simulink model "LQR-1"  (R2018a)
settings: Solver=VariableStepAuto  StartTime=0.0  StopTime=10.0  RelTol=1e-3
settings Model: Creator=86153  LastModifiedBy=86153

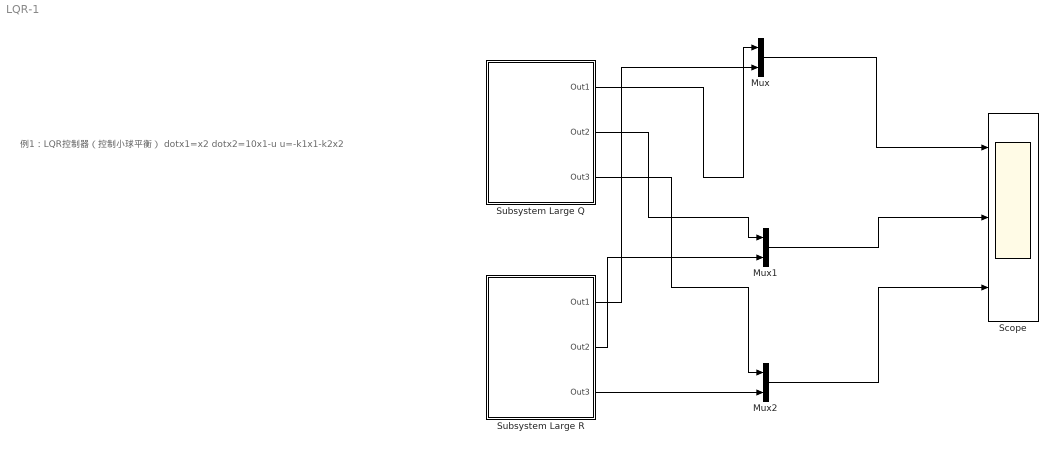
== system LQR-1 ==
  note: 例1：LQR控制器（控制小球平衡）
      | dotx1=x2
      | dotx2=10x1-u
      | u=-k1x1-k2x2
  Mux : Mux  Inputs=2
  Mux1 : Mux  Inputs=2
  Mux2 : Mux  Inputs=2
  Scope : Scope  NumInputPorts=3
  Subsystem Large Q : Subsystem
  Subsystem Large R : Subsystem
  wires:
  Subsystem Large Q/1(Out1) -> Mux/1
  Subsystem Large Q/2(Out2) -> Mux1/1
  Subsystem Large Q/3(Out3) -> Mux2/1
  Mux1/1 -> Scope/2
  Mux/1 -> Scope/1
  Mux2/1 -> Scope/3
  Subsystem Large R/1(Out1) -> Mux/2
  Subsystem Large R/2(Out2) -> Mux1/2
  Subsystem Large R/3(Out3) -> Mux2/2

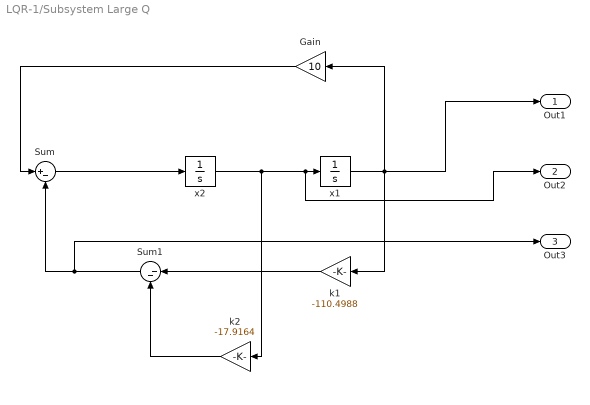
== system LQR-1/Subsystem Large Q ==
  Gain : Gain  Gain=10
  Sum : Sum  Inputs=|+-
  Sum1 : Sum  Inputs=|--
  k1 : Gain  Gain=-110.4988
  k2 : Gain  Gain=-17.9164
  x1 : Integrator  InitialCondition=5
  x2 : Integrator
  Out1 : Outport
  Out2 : Outport  Port=2
  Out3 : Outport  Port=3
  wires:
  Sum/1 -> x2/1
  x2/1 -> k2/1, Out2/1, x1/1
  x1/1 -> Out1/1, Gain/1, k1/1
  Sum1/1 -> Out3/1, Sum/2
  Gain/1 -> Sum/1
  k2/1 -> Sum1/2
  k1/1 -> Sum1/1

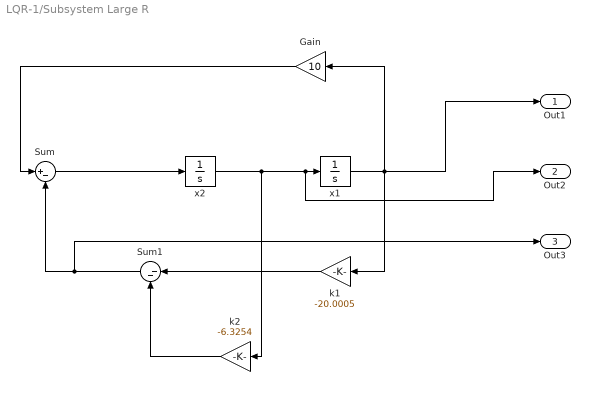
== system LQR-1/Subsystem Large R ==
  Gain : Gain  Gain=10
  Sum : Sum  Inputs=|+-
  Sum1 : Sum  Inputs=|--
  k1 : Gain  Gain=-20.0005
  k2 : Gain  Gain=-6.3254
  x1 : Integrator  InitialCondition=5
  x2 : Integrator
  Out1 : Outport
  Out2 : Outport  Port=2
  Out3 : Outport  Port=3
  wires:
  k1/1 -> Sum1/1
  k2/1 -> Sum1/2
  Gain/1 -> Sum/1
  Sum1/1 -> Sum/2, Out3/1
  x1/1 -> k1/1, Gain/1, Out1/1
  x2/1 -> x1/1, Out2/1, k2/1
  Sum/1 -> x2/1
